simulink model "daolibaixt2l"  (Simulink 8.0)
settings: Solver=ode45  StartTime=0.0  StopTime=8  MinStep=1e-3  RelTol=1e-3
libraries: fuzblock x1
settings Model: Creator=fangzhen  LastModifiedBy=fangzhen
settings SolverCC: ZeroCrossControl=DisableAll
settings DataIOCC: SignalLoggingSaveFormat=ModelDataLogs
settings DebuggingCC: FcnCallInpInsideContextMsg=EnableAllAsWarning

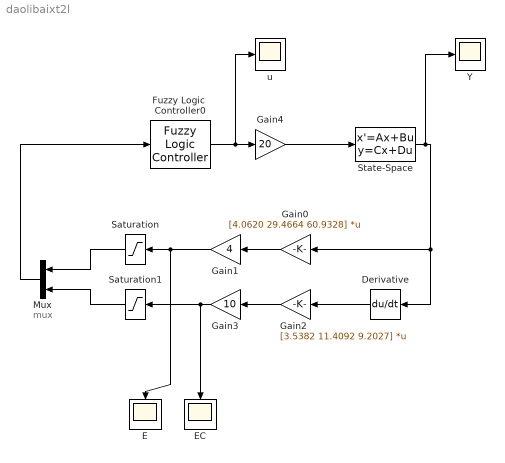
== system daolibaixt2l ==
  note: mux
  Derivative : Derivative
  E : Scope
      settings: SaveName=ScopeData2
  EC : Scope
  Fuzzy Logic  Controller0 : fuzblock/Fuzzy Logic  Controller  fis=daolibai2l
  Gain0 : Gain  Gain=[4.0620 29.4664 60.9328]  Multiplication=Matrix(K*u)
  Gain1 : Gain  Gain=4
  Gain2 : Gain  Gain=[3.5382 11.4092 9.2027]  Multiplication=Matrix(K*u)
  Gain3 : Gain  Gain=10
  Gain4 : Gain  Gain=20
  Mux : Mux  Inputs=2
  Saturation : Saturate  UpperLimit=3  LowerLimit=-3
  Saturation1 : Saturate  UpperLimit=3  LowerLimit=-3
  State-Space : StateSpace  A=[0 0 0 1 0 0;0 0 0 0 1 0;0 0 0 0 0 1;0 -2.569 0.16408 -16.667 0.01718 -0.0011;0 29.919 -15.181 40.317 -0.28268 0.0959;0 -36.656 65.378 -49.395 0.64301 -0.41489]  B=[0;0;0;8.6462;-20.914;25.642]  C=[1 0 0 0 0 0; 0 1 0 0 0 0; 0 0 1 0 0 0]  D=[0;0;0]  X0=[0.1;-0.1;0.1;0;0;0]
  Y : Scope
      settings: YMin=-0.03  YMax=0.025
  u : Scope
      settings: SaveName=ScopeData3
  wires:
  State-Space/1 -> Derivative/1, Gain0/1, Y/1
  Gain0/1 -> Gain1/1
  Fuzzy Logic  Controller0/1 -> Gain4/1, u/1
  Gain1/1 -> Saturation/1, E/1
  Gain4/1 -> State-Space/1
  Derivative/1 -> Gain2/1
  Gain2/1 -> Gain3/1
  Gain3/1 -> EC/1, Saturation1/1
  Mux/1 -> Fuzzy Logic  Controller0/1
  Saturation1/1 -> Mux/2
  Saturation/1 -> Mux/1
